simulink model "MBD_Unit_Delay"  (R2021b)
settings: Solver=FixedStepDiscrete  StartTime=0.0  StopTime=10.0  FixedStep=0.5  RelTol=1e-3
settings Model: Creator=waleed.elshemy  LastModifiedBy=waleed.elshemy
settings OptimizationCC: DefaultParameterBehavior=Inlined  UseDivisionForNetSlopeComputation=on  GainParamInheritBuiltInType=on  UseFloatMulNetSlope=on  InlineInvariantSignals=on  PassReuseOutputArgsAs=Individual arguments  ZeroExternalMemoryAtStartup=off  ZeroInternalMemoryAtStartup=off  NoFixptDivByZeroProtection=on  EfficientFloat2IntCast=on  LifeSpan=1  OptimizeBlockOrder=speed  DifferentSizesBufferReuse=on  EfficientTunableParamExpr=on
settings DebuggingCC: ParameterTunabilityLossMsg=error
settings HardwareCC: ProdLongLongMode=on
settings SFSimCC: MATLABDynamicMemAlloc=off
settings RTWCC: Description=Embedded Coder  SystemTargetFile=ert.tlc  TemplateMakefile=ert_default_tmf
settings CodeAppCC: ForceParamTrailComments=on  IgnoreCustomStorageClasses=off  OperatorAnnotations=on  SimulinkDataObjDesc=on  SFDataObjDesc=on  CustomSymbolStrGlobalVar=rt$N$M  CustomSymbolStrType=$N$M  CustomSymbolStrFcn=$N$M$F  CustomSymbolStrMacro=$N$M  InsertBlockDesc=on
settings ERTTargetCC: TargetLangStandard=C99 (ISO)  GenerateSampleERTMain=on  IncludeMdlTerminateFcn=off  CombineSignalStateStructs=on  SuppressErrorStatus=on  SupportAbsoluteTime=off  SupportComplex=off  InlinedParameterPlacement=NonHierarchical  ERTCustomFileTemplate=example_file_process.tlc  ERTFilePackagingFormat=CompactWithDataFile

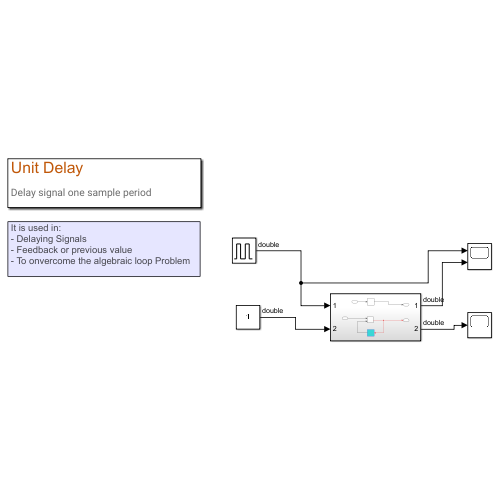
[thumbnail: Simulink's stored preview of the top-level diagram]
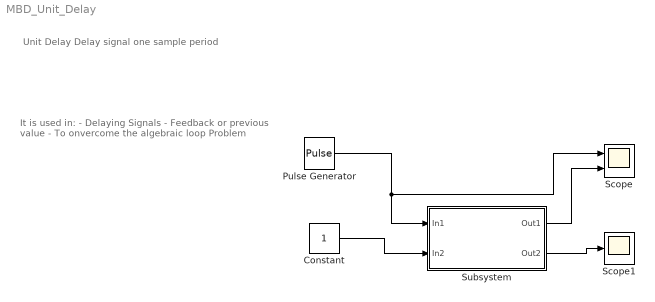
== system MBD_Unit_Delay ==
  note: It is used in:
      | - Delaying Signals
      | - Feedback or previous value
      | - To onvercome the algebraic loop Problem
  note: Unit Delay
      | Delay signal one sample period
  Constant : Constant
  Pulse Generator : DiscretePulseGenerator  PulseType=Time based  PulseWidth=25
  Scope : Scope  NumInputPorts=2
  Scope1 : Scope
  Subsystem : Subsystem
  wires:
  Pulse Generator/1 -> Subsystem/1(In1), Scope/1
  Constant/1 -> Subsystem/2(In2)
  Subsystem/1(Out1) -> Scope/2
  Subsystem/2(Out2) -> Scope1/1

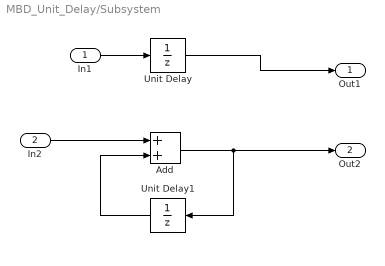
== system MBD_Unit_Delay/Subsystem ==
  In1 : Inport
  In2 : Inport  Port=2
  Add : Sum
  Unit Delay : UnitDelay  SampleTime=-1  HasFrameUpgradeWarning=on
  Unit Delay1 : UnitDelay  SampleTime=-1  HasFrameUpgradeWarning=on
  Out1 : Outport
  Out2 : Outport  Port=2
  wires:
  Add/1 -> Out2/1, Unit Delay1/1
  Unit Delay1/1 -> Add/2
  In2/1 -> Add/1
  Unit Delay/1 -> Out1/1
  In1/1 -> Unit Delay/1
